simulink model "VB_RIFKF_GNSS_INS25"  (R2023a)
settings: Solver=FixedStepAuto  StartTime=0  StopTime=500  FixedStep=0.01  RelTol=1e-3
InitFcn:
  | resilient_initNavigation1216;
  | init_param;
undefined symbols (not defined in the file or in its folder): dt, g0, gam0_rad, ISUS_flag, magnitude, p, P0, P0_RIEKF, param, pd0, pe0, phi0_rad, pn0, psi, psi0_rad, state_dim, vd0, ve0, vn0
libraries: simulink_extras x68, dspstat3 x54, sharedtransform x47, simulink x43, matrix_library x9, sharedTrackingLibrary x5, dspfactors x4, aerolibconvert2 x3, aerolibtransform2 x3
(part 21 of 22)

== matlab function VB_RIFKF_GNSS_INS25/No.1_Sensor_Data_Process1/Magn_Data_Process/MATLAB Function1 ==
  data: u input; y output
function y = Normalization(u)
   dim = 3;
   y = zeros(dim,1);
y = double(u/sqrt(u(1)^2 + u(2)^2 + u(3)^2));

== matlab function VB_RIFKF_GNSS_INS25/No.1_Sensor_Data_Process1/Magn_Data_Process/Magn_preprocessing/MATLAB Function1 ==
  data: curr_input input single; curr_output output single; sample_freq input single; cutoff_freq input single
function curr_output = second_LPF_Butter_x(curr_input,sample_freq,cutoff_freq)
   persistent input_x;
   persistent output_x;

   if isempty(input_x)
       input_x = [0;0;0];
   end
   
   if isempty(output_x)
       output_x = [0;0;0];
   end
    B = [0,0,0];
    A = [0,0,0];
    M_PI_F = 3.1415926;
	fr = sample_freq / cutoff_freq;
	ohm = tan( M_PI_F / fr );
	c = 1.0 + 2.0 * cos( M_PI_F / 4.0 ) * ohm + ohm * ohm;
	B(1) = ohm * ohm / c;
	B(2) = 2.0 * B(1);
	B(3) = B(1);
	A(1) = 2.0 * ( ohm * ohm - 1.0) / c;
	A(2) = (1.0 - 2.0 * cos( M_PI_F / 4.0 ) * ohm + ohm * ohm) / c;
	%/*获取最新输入*/
	input_x(3) = curr_input;
	%/* Butterworth */
	output_x(3) =B(1) * input_x(3) + B(2) * input_x(2) +B(3) * input_x(1) - A(1) * output_x(2) - A(2) * output_x(1);
	curr_output = single(output_x(3));
   % /* 输入序列保存 */
	input_x(1) = input_x(2);
	input_x(2) = input_x(3);
	%/*输出序列保存 */
	output_x(1) = output_x(2);
	output_x(2) = output_x(3);

== matlab function VB_RIFKF_GNSS_INS25/No.1_Sensor_Data_Process1/Magn_Data_Process/Magn_preprocessing/MATLAB Function2 ==
  data: curr_input input single; curr_output output single; sample_freq input single; cutoff_freq input single
function curr_output = second_LPF_Butter_x(curr_input,sample_freq,cutoff_freq)
   persistent input_x;
   persistent output_x;

   if isempty(input_x)
       input_x = [0;0;0];
   end
   
   if isempty(output_x)
       output_x = [0;0;0];
   end
    B = [0,0,0];
    A = [0,0,0];
    M_PI_F = 3.1415926;
	fr = sample_freq / cutoff_freq;
	ohm = tan( M_PI_F / fr );
	c = 1.0 + 2.0 * cos( M_PI_F / 4.0 ) * ohm + ohm * ohm;
	B(1) = ohm * ohm / c;
	B(2) = 2.0 * B(1);
	B(3) = B(1);
	A(1) = 2.0 * ( ohm * ohm - 1.0) / c;
	A(2) = (1.0 - 2.0 * cos( M_PI_F / 4.0 ) * ohm + ohm * ohm) / c;
	%/*获取最新输入*/
	input_x(3) = curr_input;
	%/* Butterworth */
	output_x(3) =B(1) * input_x(3) + B(2) * input_x(2) +B(3) * input_x(1) - A(1) * output_x(2) - A(2) * output_x(1);
	curr_output = single(output_x(3));
   % /* 输入序列保存 */
	input_x(1) = input_x(2);
	input_x(2) = input_x(3);
	%/*输出序列保存 */
	output_x(1) = output_x(2);
	output_x(2) = output_x(3);

== matlab function VB_RIFKF_GNSS_INS25/No.1_Sensor_Data_Process1/Magn_Data_Process/Magn_preprocessing/MATLAB Function3 ==
  data: curr_input input single; curr_output output single; sample_freq input single; cutoff_freq input single
function curr_output = second_LPF_Butter_x(curr_input,sample_freq,cutoff_freq)
   persistent input_x;
   persistent output_x;

   if isempty(input_x)
       input_x = [0;0;0];
   end
   
   if isempty(output_x)
       output_x = [0;0;0];
   end
    B = [0,0,0];
    A = [0,0,0];
    M_PI_F = 3.1415926;
	fr = sample_freq / cutoff_freq;
	ohm = tan( M_PI_F / fr );
	c = 1.0 + 2.0 * cos( M_PI_F / 4.0 ) * ohm + ohm * ohm;
	B(1) = ohm * ohm / c;
	B(2) = 2.0 * B(1);
	B(3) = B(1);
	A(1) = 2.0 * ( ohm * ohm - 1.0) / c;
	A(2) = (1.0 - 2.0 * cos( M_PI_F / 4.0 ) * ohm + ohm * ohm) / c;
	%/*获取最新输入*/
	input_x(3) = curr_input;
	%/* Butterworth */
	output_x(3) =B(1) * input_x(3) + B(2) * input_x(2) +B(3) * input_x(1) - A(1) * output_x(2) - A(2) * output_x(1);
	curr_output =single(output_x(3));
   % /* 输入序列保存 */
	input_x(1) = input_x(2);
	input_x(2) = input_x(3);
	%/*输出序列保存 */
	output_x(1) = output_x(2);
	output_x(2) = output_x(3);

== matlab function VB_RIFKF_GNSS_INS25/No.1_Sensor_Data_Process1/Subsystem/TD_baro/MATLAB Function2 ==
  data: T input single; u1 output; u0 input; u1 input single; u2 input single; h input single; r input single; u2 output
function [u1,u2]=diff_TD_2(T,u0,u1,u2,h,r)
    %init
    %T是信号周期，u0原始信号输入，u1跟踪原始信号，u2原始信号差分值，
    %h滤波因子（h=T时接近一阶差分）越大滤波好延迟大；r速度因子，越大跟踪的越快但是噪声放大；

	x1=0; x2=0;
	delta=0;
	delta0=0;
	y=0;
	fabs_y=0;
	a0=0;
	a=0;
    fst=0;
    
	x1 = u1;
	x2 = u2;
	delta = r*h;
	delta0 = delta*h;
	y = x1 - u0 + h*x2;
	fabs_y = abs(y);   
	a0 = sqrt(delta*delta + 8 * r*fabs_y);
    
	if (fabs_y <= delta0)
		a = x2 + y / h;
    else
        a = x2 + 0.5*(a0 - delta)*sign(y);
    end
    
	if (abs(a) <= delta)
		fst = -r*a / delta;
    else
		fst = -r*sign(a);
    end
	u1 = single(x1 + T*x2); %计算跟踪信号
	u2 = single(x2 + T*fst); % 计算微分信号

== matlab function VB_RIFKF_GNSS_INS25/ISUS_RIEKF3/Error State Kalman Filter M3/MATLAB Function4 ==
  data: t input; u input; y output
function y = fcn(t,u)
if  t<300
    y = u;
elseif t<400 
    y = false;
else 
    y = u;
end

== matlab function VB_RIFKF_GNSS_INS25/No.1_Sensor_Data_Process1/TOF_Data_Process/TD_baro/MATLAB Function2 ==
  data: T input single; u1 output; u0 input; u1 input single; u2 input single; h input single; r input single; u2 output
function [u1,u2]=diff_TD_2(T,u0,u1,u2,h,r)
    %init
    %T是信号周期，u0原始信号输入，u1跟踪原始信号，u2原始信号差分值，
    %h滤波因子（h=T时接近一阶差分）越大滤波好延迟大；r速度因子，越大跟踪的越快但是噪声放大；

	x1=0; x2=0;
	delta=0;
	delta0=0;
	y=0;
	fabs_y=0;
	a0=0;
	a=0;
    fst=0;
    
	x1 = u1;
	x2 = u2;
	delta = r*h;
	delta0 = delta*h;
	y = x1 - u0 + h*x2;
	fabs_y = abs(y);   
	a0 = sqrt(delta*delta + 8 * r*fabs_y);
    
	if (fabs_y <= delta0)
		a = x2 + y / h;
    else
        a = x2 + 0.5*(a0 - delta)*sign(y);
    end
    
	if (abs(a) <= delta)
		fst = -r*a / delta;
    else
		fst = -r*sign(a);
    end
	u1 = single(x1 + T*x2); %计算跟踪信号
	u2 = single(x2 + T*fst); % 计算微分信号

== matlab function VB_RIFKF_GNSS_INS25/read FC1_/MATLAB Function ==
  data: dpsi input; y output
function y = wrap_dpsi(dpsi)
    if dpsi > 180
        dpsi = dpsi -360;
    elseif dpsi < -180
        dpsi = dpsi + 360;
    else 
        dpsi = dpsi;
    end
y = dpsi;

== matlab function VB_RIFKF_GNSS_INS25/No.1_Sensor_Data_Process1/baro_Data_Process/TD_baro/MATLAB Function2 ==
  data: T input single; u1 output; u0 input; u1 input single; u2 input single; h input single; r input single; u2 output
function [u1,u2]=diff_TD_2(T,u0,u1,u2,h,r)
    %init
    %T是信号周期，u0原始信号输入，u1跟踪原始信号，u2原始信号差分值，
    %h滤波因子（h=T时接近一阶差分）越大滤波好延迟大；r速度因子，越大跟踪的越快但是噪声放大；

	x1=0; x2=0;
	delta=0;
	delta0=0;
	y=0;
	fabs_y=0;
	a0=0;
	a=0;
    fst=0;
    
	x1 = u1;
	x2 = u2;
	delta = r*h;
	delta0 = delta*h;
	y = x1 - u0 + h*x2;
	fabs_y = abs(y);   
	a0 = sqrt(delta*delta + 8 * r*fabs_y);
    
	if (fabs_y <= delta0)
		a = x2 + y / h;
    else
        a = x2 + 0.5*(a0 - delta)*sign(y);
    end
    
	if (abs(a) <= delta)
		fst = -r*a / delta;
    else
		fst = -r*sign(a);
    end
	u1 = single(x1 + T*x2); %计算跟踪信号
	u2 = single(x2 + T*fst); % 计算微分信号

== matlab function VB_RIFKF_GNSS_INS25/ISUS_RIEKF3/Error State Kalman Filter M1/MATLAB Function4 ==
  data: t input; y output
function y = fcn(t)
if t<200 
    y = 0;
elseif t<300
    y=1;

elseif t<400
    y=0;
else 
    y=0;
end

end

== matlab function VB_RIFKF_GNSS_INS25/ISUS_RIEKF2/Error State Kalman Filter M1/Cal Q1/MATLAB Function1 ==
  data: Q output; dt input
function Q = fcn(dt)
    % G.block(0, 0, 3, 3) = -exp_so3(-w_hat * dt) * Jr_so3(-w_hat * dt) * dt;
    %    G.block(6, 3, 3, 3) = -R_Gtoi.transpose() * dt;
    %    G.block(3, 3, 3, 3) = -0.5 * R_Gtoi.transpose() * dt * dt;
    %    G.block(9, 6, 3, 3).setIdentity();
    %    G.block(12, 9, 3, 3).setIdentity();
    

    cov_dim = 12;
    Q = zeros(cov_dim,cov_dim);
%     noises_sigma_a_2 = 2.0000e-4^2;
%     noises_sigma_w_2 = 1.6968e-4^2;
%     noises_sigma_ab_2 = 3.0000e-4^2;
%     noises_sigma_wb_2 = 1.9393e-5^2;
    noises_sigma_a_2 = 0.001^2*1;
    %noises_sigma_w_2 = 0.0001^2;
    noises_sigma_w_2 = 0.00001^2;
    noises_sigma_ab_2 = 1.0000e-4^2*1;
    noises_sigma_wb_2 = 0.0002^2;
    % noises_sigma_mb_2 = 0.001^2;
    % noises_sigma_dtheta_2 = (1/57.3)^2;
    % noises_sigma_dwind_2 = 0.01^2;
    Q = diag([noises_sigma_w_2 / dt * ones(3,1); ...
                noises_sigma_a_2 / dt * ones(3,1); ...
                noises_sigma_wb_2 * dt * ones(3,1); ...
                noises_sigma_ab_2 * dt * ones(3,1); ...
                ]);
    

end

== matlab function VB_RIFKF_GNSS_INS25/read FC1_1/MATLAB Function ==
  data: dpsi input; y output
function y = wrap_dpsi(dpsi)
    if dpsi > 180
        dpsi = dpsi -360;
    elseif dpsi < -180
        dpsi = dpsi + 360;
    else 
        dpsi = dpsi;
    end
y = dpsi;

== matlab function VB_RIFKF_GNSS_INS25/No.1_Sensor_Data_Process2/GPS_Data_Process/LLA2NED/initGPSLLA ==
  data: QGCinitflag input; gpsLLA0_rad output; GPSfixtype input; gps_LLA_rad input; init_GPSLLAflag output
function [gpsLLA0_rad,init_GPSLLAflag] = initGPSLLA0(QGCinitflag,GPSfixtype,gps_LLA_rad)
    persistent initGPSLLAflag;
    persistent gpsLLA0;

    if isempty(initGPSLLAflag)
        initGPSLLAflag = 0;
    end
    if isempty(gpsLLA0)
        %初始GPS未进入定位状态，给定值
%          gpsLLA0 = [28.2/57.3;113/57.3;0];
        gpsLLA0 = zeros(3,1);
    end
    if (initGPSLLAflag == 0 && GPSfixtype >= 1) || (QGCinitflag == 1 && GPSfixtype >= 1)
        % 当GPS第一次初始化位置时，当GPSfixtype >=1 时，自动初始化一次位置，initGPSLLAflag置1
        % 或者是利用QGCinitflag地面站重新修正，不过需要满足GPSfixtype>=1的条件
        gpsLLA0 = gps_LLA_rad;
        initGPSLLAflag = 1;
    end
    gpsLLA0_rad = gpsLLA0;
    init_GPSLLAflag = initGPSLLAflag;
end

== matlab function VB_RIFKF_GNSS_INS25/No.1_Sensor_Data_Process2/IMU_Data_Process/accl_preprocessing2/MATLAB Function1 ==
  data: curr_input input; curr_output output single; sample_freq input; cutoff_freq input
function curr_output = second_LPF_Butter_x(curr_input,sample_freq,cutoff_freq)
   persistent input_x;
   persistent output_x;

   if isempty(input_x)
       input_x = [0;0;0];
   end
   
   if isempty(output_x)
       output_x = [0;0;0];
   end
    B = [0,0,0];
    A = [0,0,0];
    M_PI_F = 3.1415926;
	fr = sample_freq / cutoff_freq;
	ohm = tan( M_PI_F / fr );
	c = 1.0 + 2.0 * cos( M_PI_F / 4.0 ) * ohm + ohm * ohm;
	B(1) = ohm * ohm / c;
	B(2) = 2.0 * B(1);
	B(3) = B(1);
	A(1) = 2.0 * ( ohm * ohm - 1.0) / c;
	A(2) = (1.0 - 2.0 * cos( M_PI_F / 4.0 ) * ohm + ohm * ohm) / c;
	%/*获取最新输入*/
	input_x(3) = curr_input;
	%/* Butterworth */
	output_x(3) =B(1) * input_x(3) + B(2) * input_x(2) +B(3) * input_x(1) - A(1) * output_x(2) - A(2) * output_x(1);
	curr_output = single(output_x(3));
   % /* 输入序列保存 */
	input_x(1) = input_x(2);
	input_x(2) = input_x(3);
	%/*输出序列保存 */
	output_x(1) = output_x(2);
	output_x(2) = output_x(3);

== matlab function VB_RIFKF_GNSS_INS25/ISUS_RIEKF3/INS propogation1/att update/MATLAB Function ==
  data: Rbn_k_1 input; Rbn output; w input; dt input
function Rbn = fcn(Rbn_k_1, w, dt)
    Rbn =  Rbn_k_1 * exp_so3( w * dt);
end

== matlab function VB_RIFKF_GNSS_INS25/ISUS_RIEKF3/Error State Kalman Filter M1/VB-Extended Kalman Filter M2/Correct M1/MATLAB Function ==
  data: u input; y output
function y = fcn(u)

y = tril(u);

== matlab function VB_RIFKF_GNSS_INS25/No.1_Sensor_Data_Process2/IMU_Data_Process/accl_preprocessing2/MATLAB Function2 ==
  data: curr_input input; curr_output output single; sample_freq input; cutoff_freq input
function curr_output = second_LPF_Butter_x(curr_input,sample_freq,cutoff_freq)
   persistent input_x;
   persistent output_x;

   if isempty(input_x)
       input_x = [0;0;0];
   end
   
   if isempty(output_x)
       output_x = [0;0;0];
   end
    B = [0,0,0];
    A = [0,0,0];
    M_PI_F = 3.1415926;
	fr = sample_freq / cutoff_freq;
	ohm = tan( M_PI_F / fr );
	c = 1.0 + 2.0 * cos( M_PI_F / 4.0 ) * ohm + ohm * ohm;
	B(1) = ohm * ohm / c;
	B(2) = 2.0 * B(1);
	B(3) = B(1);
	A(1) = 2.0 * ( ohm * ohm - 1.0) / c;
	A(2) = (1.0 - 2.0 * cos( M_PI_F / 4.0 ) * ohm + ohm * ohm) / c;
	%/*获取最新输入*/
	input_x(3) = curr_input;
	%/* Butterworth */
	output_x(3) =B(1) * input_x(3) + B(2) * input_x(2) +B(3) * input_x(1) - A(1) * output_x(2) - A(2) * output_x(1);
	curr_output = single(output_x(3));
   % /* 输入序列保存 */
	input_x(1) = input_x(2);
	input_x(2) = input_x(3);
	%/*输出序列保存 */
	output_x(1) = output_x(2);
	output_x(2) = output_x(3);

== matlab function VB_RIFKF_GNSS_INS25/No.1_Sensor_Data_Process2/IMU_Data_Process/accl_preprocessing2/MATLAB Function3 ==
  data: curr_input input; curr_output output single; sample_freq input; cutoff_freq input
function curr_output = second_LPF_Butter_x(curr_input,sample_freq,cutoff_freq)
   persistent input_x;
   persistent output_x;

   if isempty(input_x)
       input_x = [0;0;0];
   end
   
   if isempty(output_x)
       output_x = [0;0;0];
   end
    B = [0,0,0];
    A = [0,0,0];
    M_PI_F = 3.1415926;
	fr = sample_freq / cutoff_freq;
	ohm = tan( M_PI_F / fr );
	c = 1.0 + 2.0 * cos( M_PI_F / 4.0 ) * ohm + ohm * ohm;
	B(1) = ohm * ohm / c;
	B(2) = 2.0 * B(1);
	B(3) = B(1);
	A(1) = 2.0 * ( ohm * ohm - 1.0) / c;
	A(2) = (1.0 - 2.0 * cos( M_PI_F / 4.0 ) * ohm + ohm * ohm) / c;
	%/*获取最新输入*/
	input_x(3) = curr_input;
	%/* Butterworth */
	output_x(3) =B(1) * input_x(3) + B(2) * input_x(2) +B(3) * input_x(1) - A(1) * output_x(2) - A(2) * output_x(1);
	curr_output = single(output_x(3));
   % /* 输入序列保存 */
	input_x(1) = input_x(2);
	input_x(2) = input_x(3);
	%/*输出序列保存 */
	output_x(1) = output_x(2);
	output_x(2) = output_x(3);

== matlab function VB_RIFKF_GNSS_INS25/No.1_Sensor_Data_Process2/IMU_Data_Process/gyro_preprocessing2/MATLAB Function1 ==
  data: curr_input input single; curr_output output single; sample_freq input single; cutoff_freq input single
function curr_output = second_LPF_Butter_x(curr_input,sample_freq,cutoff_freq)
   persistent input_x;
   persistent output_x;

   if isempty(input_x)
       input_x = [0;0;0];
   end
   
   if isempty(output_x)
       output_x = [0;0;0];
   end
    B = [0,0,0];
    A = [0,0,0];
    M_PI_F = 3.1415926;
	fr = sample_freq / cutoff_freq;
	ohm = tan( M_PI_F / fr );
	c = 1.0 + 2.0 * cos( M_PI_F / 4.0 ) * ohm + ohm * ohm;
	B(1) = ohm * ohm / c;
	B(2) = 2.0 * B(1);
	B(3) = B(1);
	A(1) = 2.0 * ( ohm * ohm - 1.0) / c;
	A(2) = (1.0 - 2.0 * cos( M_PI_F / 4.0 ) * ohm + ohm * ohm) / c;
	%/*获取最新输入*/
	input_x(3) = curr_input;
	%/* Butterworth */
	output_x(3) =B(1) * input_x(3) + B(2) * input_x(2) +B(3) * input_x(1) - A(1) * output_x(2) - A(2) * output_x(1);
	curr_output = single(output_x(3));
   % /* 输入序列保存 */
	input_x(1) = input_x(2);
	input_x(2) = input_x(3);
	%/*输出序列保存 */
	output_x(1) = output_x(2);
	output_x(2) = output_x(3);

== matlab function VB_RIFKF_GNSS_INS25/ISUS_RIEKF3/Error State Kalman Filter M1/VB-Extended Kalman Filter M2/Correct M1/Subsystem2/MATLAB Function1 ==
  data: u input; y output; X input; ISUS_flag input
function y = fcn(u, X, ISUS_flag)
if ISUS_flag == 0
    y = X;
else
     y = u;
    %y(1:9,1:9) = u;
end

== matlab function VB_RIFKF_GNSS_INS25/ISUS_RIEKF3/Error State Kalman Filter M1/VB-Extended Kalman Filter M2/Correct M1/innovation calculation/MATLAB Function ==
  data: u input; y output
function y = fcn(u)

y = u*u';

== matlab function VB_RIFKF_GNSS_INS25/ISUS_RIEKF3/Error State Kalman Filter M1/VB-Extended Kalman Filter M2/Output/MATLAB Function ==
  data: S input; P output
function P = fcn(S)
    
    % Get back Covariance from Square-root Covariance
    P = S*S';
    %P = 1/2*(S+S');
    
end

== matlab function VB_RIFKF_GNSS_INS25/No.1_Sensor_Data_Process2/IMU_Data_Process/gyro_preprocessing2/MATLAB Function2 ==
  data: curr_input input single; curr_output output single; sample_freq input single; cutoff_freq input single
function curr_output = second_LPF_Butter_x(curr_input,sample_freq,cutoff_freq)
   persistent input_x;
   persistent output_x;

   if isempty(input_x)
       input_x = [0;0;0];
   end
   
   if isempty(output_x)
       output_x = [0;0;0];
   end
    B = [0,0,0];
    A = [0,0,0];
    M_PI_F = 3.1415926;
	fr = sample_freq / cutoff_freq;
	ohm = tan( M_PI_F / fr );
	c = 1.0 + 2.0 * cos( M_PI_F / 4.0 ) * ohm + ohm * ohm;
	B(1) = ohm * ohm / c;
	B(2) = 2.0 * B(1);
	B(3) = B(1);
	A(1) = 2.0 * ( ohm * ohm - 1.0) / c;
	A(2) = (1.0 - 2.0 * cos( M_PI_F / 4.0 ) * ohm + ohm * ohm) / c;
	%/*获取最新输入*/
	input_x(3) = curr_input;
	%/* Butterworth */
	output_x(3) =B(1) * input_x(3) + B(2) * input_x(2) +B(3) * input_x(1) - A(1) * output_x(2) - A(2) * output_x(1);
	curr_output = single(output_x(3));
   % /* 输入序列保存 */
	input_x(1) = input_x(2);
	input_x(2) = input_x(3);
	%/*输出序列保存 */
	output_x(1) = output_x(2);
	output_x(2) = output_x(3);

== matlab function VB_RIFKF_GNSS_INS25/ISUS_RIEKF3/Error State Kalman Filter M1/VB-Extended Kalman Filter M2/Predict/Predict ==
  settings: updateMethod=DISCRETE  sampleTime=SampleTime
  data: x input; xNew output; P input; Q input; uState input; unused input; P output; pS parameter
function [xNew,P] = fcn(x,P,Q,uState,~,pS)
% ekfCorrect Prediction step for EKF
%
%   Copyright 2016-2021 The MathWorks, Inc.

%#codegen

% If process noise is time-varying then compute square-root
% factorization.
if pS.HasTimeVaryingQ
   Q = matlabshared.tracking.internal.svdPSD(Q);
end

% Construct fcn handles
if pS.IsSimulinkFcn
    StateTransitionJacobianFcnH_SL = str2func(pS.FcnName);
    if pS.HasAdditiveNoise
        StateTransitionFcnH = @(fState)StateTransitionJacobianFcnH_SL(fState);
    else
        StateTransitionFcnH = @(fState,fProcNoise)StateTransitionJacobianFcnH_SL(fState,fProcNoise);
    end
else
    StateTransitionFcnH = str2func(pS.FcnName);
end
if pS.HasJacobian
    if pS.IsSimulinkFcn
        StateTransitionJacobianFcnH_SL = str2func(pS.JacobianFcnName);
        if pS.HasAdditiveNoise
            StateTransitionJacobianFcnH = @(fState)StateTransitionJacobianFcnH_SL(fState);
        else
            StateTransitionJacobianFcnH = @(fState,fProcNoise)StateTransitionJacobianFcnH_SL(fState,fProcNoise);
        end
    else
        StateTransitionJacobianFcnH = str2func(pS.JacobianFcnName);
    end
else
    StateTransitionJacobianFcnH = [];
end

switch pS.NumberOfExtraArgumentInports
    case 0
        extraArgs = {};
    case 1
        extraArgs = {uState};
    otherwise
        assert(false);
end

% Check if dimensions and type of State and Jacobian are correct
if pS.HasAdditiveNoise
   % Additive noise
   
   % StateTransitionFcn
   xTry = StateTransitionFcnH(x, extraArgs{:});
   
   if pS.IsSimulinkFcn
      hasError = any(size(x) ~= size(xTry));
   else
      hasError = any(size(x) ~= size(xTry)) || ~isa(xTry, class(x));
   end
   
   coder.internal.errorIf(...
      hasError,...
      'shared_tracking:ExtendedKalmanFilter:StateNonMatchingSizeOrClass',...
      'StateTransitionFcn', 'State', numel(x));
   
   if pS.HasJacobian
      % Jacobian
      F = StateTransitionJacobianFcnH(x, extraArgs{:});
      % F needs to be square
      isSizeNotCorrect = ~all(size(F) == numel(x));
      
      if pS.IsSimulinkFcn
         hasError = isSizeNotCorrect;
      else
         hasError = isSizeNotCorrect || ~isa(F, class(x));
      end
      
      coder.internal.errorIf(...
         hasError,...
         'shared_tracking:ExtendedKalmanFilter:StateTransitionJacobianNonMatchingSizeOrClass',...
         'StateTransitionJacobianFcn', numel(x));
   end
else
   % Non-additive noise
   
   % StateTransitionFcn
   xTry = StateTransitionFcnH(x, zeros(size(Q,1),1,'like',x),extraArgs{:});
   
   if pS.IsSimulinkFcn
      hasError = any(size(x) ~= size(xTry));
   else
      hasError = any(size(x) ~= size(xTry)) || ~isa(xTry, class(x));
   end
   
   coder.internal.errorIf(...
      hasError,...
      'shared_tracking:ExtendedKalmanFilter:StateNonMatchingSizeOrClass',...
      'StateTransitionFcn', 'State', numel(x))
   
   if pS.HasJacobian
      % Jacobian
      F = StateTransitionJacobianFcnH(x, zeros(size(Q,1),1,'like',x),extraArgs{:});
      % F needs to be square
      isSizeNotCorrect = ~all(size(F) == numel(x));
      
      if pS.IsSimulinkFcn
         hasError = isSizeNotCorrect;
      else
         hasError = isSizeNotCorrect || ~isa(F, class(x));
      end
       
      coder.internal.errorIf(...
         hasError,...
         'shared_tracking:ExtendedKalmanFilter:StateTransitionJacobianNonMatchingSizeOrClass',...
         'StateTransitionJacobianFcn', numel(x));
   end
end

xNew = zeros(size(x),'like',x); %#ok<PREALL>

if pS.HasAdditiveNoise
    [xNew,P] = matlabshared.tracking.internal.EKFPredictorAdditive.predict(...
        Q,x,P,StateTransitionFcnH,StateTransitionJacobianFcnH,extraArgs{:});
else    
    [xNew,P] = matlabshared.tracking.internal.EKFPredictorNonAdditive.predict(...
        Q,x,P,StateTransitionFcnH,StateTransitionJacobianFcnH,extraArgs{:});
end
end

== matlab function VB_RIFKF_GNSS_INS25/read FC1_/Subsystem/MATLAB Function ==
  data: u input; y output; u_1 input
function y = fcn(u,u_1)
if abs(u) > 100
    y = u_1;
end
y = u;

== matlab function VB_RIFKF_GNSS_INS25/No.1_Sensor_Data_Process2/IMU_Data_Process/gyro_preprocessing2/MATLAB Function3 ==
  data: curr_input input single; curr_output output single; sample_freq input single; cutoff_freq input single
function curr_output = second_LPF_Butter_x(curr_input,sample_freq,cutoff_freq)
   persistent input_x;
   persistent output_x;

   if isempty(input_x)
       input_x = [0;0;0];
   end
   
   if isempty(output_x)
       output_x = [0;0;0];
   end
    B = [0,0,0];
    A = [0,0,0];
    M_PI_F = 3.1415926;
	fr = sample_freq / cutoff_freq;
	ohm = tan( M_PI_F / fr );
	c = 1.0 + 2.0 * cos( M_PI_F / 4.0 ) * ohm + ohm * ohm;
	B(1) = ohm * ohm / c;
	B(2) = 2.0 * B(1);
	B(3) = B(1);
	A(1) = 2.0 * ( ohm * ohm - 1.0) / c;
	A(2) = (1.0 - 2.0 * cos( M_PI_F / 4.0 ) * ohm + ohm * ohm) / c;
	%/*获取最新输入*/
	input_x(3) = curr_input;
	%/* Butterworth */
	output_x(3) =B(1) * input_x(3) + B(2) * input_x(2) +B(3) * input_x(1) - A(1) * output_x(2) - A(2) * output_x(1);
	curr_output = single(output_x(3));
   % /* 输入序列保存 */
	input_x(1) = input_x(2);
	input_x(2) = input_x(3);
	%/*输出序列保存 */
	output_x(1) = output_x(2);
	output_x(2) = output_x(3);

== matlab function VB_RIFKF_GNSS_INS25/ISUS_RIEKF3/INS propogation1/att update/MATLAB Function2 ==
  data: delta input; Rbn_correct output single size=[3,3]; Rbn input
function Rbn_correct = fcn(delta, Rbn)
    Rbn_correct = zeros(3,3);
     Rbn_correct = exp_so3(delta)* Rbn;
    %Rbn_correct =( eye(3) + skewMat(delta))* Rbn;
end

== matlab function VB_RIFKF_GNSS_INS25/No.1_Sensor_Data_Process2/Magn_Data_Process/MATLAB Function1 ==
  data: u input; y output
function y = Normalization(u)
   dim = 3;
   y = zeros(dim,1);
y = double(u/sqrt(u(1)^2 + u(2)^2 + u(3)^2));

== matlab function VB_RIFKF_GNSS_INS25/No.1_Sensor_Data_Process2/Magn_Data_Process/Magn_preprocessing/MATLAB Function1 ==
  data: curr_input input single; curr_output output single; sample_freq input single; cutoff_freq input single
function curr_output = second_LPF_Butter_x(curr_input,sample_freq,cutoff_freq)
   persistent input_x;
   persistent output_x;

   if isempty(input_x)
       input_x = [0;0;0];
   end
   
   if isempty(output_x)
       output_x = [0;0;0];
   end
    B = [0,0,0];
    A = [0,0,0];
    M_PI_F = 3.1415926;
	fr = sample_freq / cutoff_freq;
	ohm = tan( M_PI_F / fr );
	c = 1.0 + 2.0 * cos( M_PI_F / 4.0 ) * ohm + ohm * ohm;
	B(1) = ohm * ohm / c;
	B(2) = 2.0 * B(1);
	B(3) = B(1);
	A(1) = 2.0 * ( ohm * ohm - 1.0) / c;
	A(2) = (1.0 - 2.0 * cos( M_PI_F / 4.0 ) * ohm + ohm * ohm) / c;
	%/*获取最新输入*/
	input_x(3) = curr_input;
	%/* Butterworth */
	output_x(3) =B(1) * input_x(3) + B(2) * input_x(2) +B(3) * input_x(1) - A(1) * output_x(2) - A(2) * output_x(1);
	curr_output = single(output_x(3));
   % /* 输入序列保存 */
	input_x(1) = input_x(2);
	input_x(2) = input_x(3);
	%/*输出序列保存 */
	output_x(1) = output_x(2);
	output_x(2) = output_x(3);

== matlab function VB_RIFKF_GNSS_INS25/ISUS_RIEKF2/Error State Kalman Filter M1/Extended Kalman Filter M1/Correct M1/Correct ==
  settings: updateMethod=DISCRETE  sampleTime=SampleTime
  data: x input; xNew output; P input; P output; yMeas input; R input; uMeas input; blockOrdering input; pM parameter; blockOrdering output
function [xNew,P,blockOrdering] = fcn(x,P,yMeas,R,uMeas,blockOrdering,pM)
% ekfCorrect Correction step for EKF
%
%   Copyright 2016-2021 The MathWorks, Inc.

%#codegen

% If measurement noise is time-varying then compute square-root
% factorization.
if pM.HasTimeVaryingR
   R = matlabshared.tracking.internal.svdPSD(R);
end

% Construct the function handle for measurement fcn
if pM.IsSimulinkFcn
    MeasurementFcnH_SL = str2func(pM.FcnName);
    if pM.HasAdditiveNoise
        MeasurementFcnH = @(fState)MeasurementFcnH_SL(fState);
    else
        MeasurementFcnH = @(fState,fMeasNoise)MeasurementFcnH_SL(fState,fMeasNoise);
    end
else
    MeasurementFcnH = str2func(pM.FcnName);
end

% Construct the function handle for measurement Jacobian fcn
if pM.HasJacobian
    if pM.IsSimulinkFcn
        MeasurementJacobianFcnH_SL = str2func(pM.JacobianFcnName);
        if pM.HasAdditiveNoise
            MeasurementJacobianFcnH = @(fState)MeasurementJacobianFcnH_SL(fState);
        else
            MeasurementJacobianFcnH = @(fState,fMeasNoise)MeasurementJacobianFcnH_SL(fState,fMeasNoise);
        end
    else
        MeasurementJacobianFcnH = str2func(pM.JacobianFcnName);
    end
else
    MeasurementJacobianFcnH = [];
end

% Handle (optional) extra input arguments of the measurement & jacobian fcns
switch pM.NumberOfExtraArgumentInports
    case 0
        extraArgs = {};
    case 1
        extraArgs = {uMeas};
    otherwise
        assert(false);
end

% Construct the corrector, perform the update
if pM.HasAdditiveNoise
    ekfCorrector = matlabshared.tracking.internal.EKFCorrectorAdditive();
else
    ekfCorrector = matlabshared.tracking.internal.EKFCorrectorNonAdditive();
end

% Check if dimensions and type of Measurement and Jacobian are correct
if pM.HasAdditiveNoise
   % Additive noise
   
   % MeasurementFcn
   ztry = MeasurementFcnH(x, extraArgs{:});
   
   if pM.IsSimulinkFcn
      hasError = (numel(ztry) ~= numel(yMeas));
   else
      hasError = (numel(ztry) ~= numel(yMeas)) || ~isa(ztry, class(x));
   end
   
   coder.internal.errorIf(...
      hasError,...
      'shared_tracking:ExtendedKalmanFilter:MeasurementNonMatchingSizeOrClass',...
      'MeasurementFcn');
   
   if pM.HasJacobian
      % MeasurementJacobianFcn
      Htry = MeasurementJacobianFcnH(x, extraArgs{:});
      isSizeNotCorrect = numel(yMeas) ~= size(Htry,1) || numel(x) ~= size(Htry,2);
      
      if pM.IsSimulinkFcn
         hasError = isSizeNotCorrect;
      else
         hasError = isSizeNotCorrect || ~isa(Htry, class(x));
      end
      
      coder.internal.errorIf(...
         hasError,...
         'shared_tracking:ExtendedKalmanFilter:MeasurementJacobianNonMatchingSizeOrClass',...
         'MeasurementJacobianFcn',numel(yMeas),numel(x));
   end   
else
   % Non-additive noise
   
   % MeasurementFcn
   ztry = MeasurementFcnH(...
      x, zeros(size(R,1),1,'like',x), ...
      extraArgs{:});   

   if pM.IsSimulinkFcn
      hasError = (numel(ztry) ~= numel(yMeas));
   else
      hasError = (numel(ztry) ~= numel(yMeas)) || ~isa(ztry, class(x));
   end
   
   coder.internal.errorIf(...
      hasError,...
      'shared_tracking:ExtendedKalmanFilter:MeasurementNonMatchingSizeOrClass',...
      'MeasurementFcn');
   
   if pM.HasJacobian
      % MeasurementJacobianFcn
      Htry = MeasurementJacobianFcnH(...
         x, zeros(size(R,1),1,'like',x), ...
         extraArgs{:});
      
      isSizeNotCorrect = numel(yMeas) ~= size(Htry,1) || numel(x) ~= size(Htry,2);     
      
      if pM.IsSimulinkFcn
         hasError = isSizeNotCorrect;
      else
         hasError = isSizeNotCorrect || ~isa(Htry, class(x));
      end
      
      coder.internal.errorIf(...
         hasError,...
         'shared_tracking:ExtendedKalmanFilter:MeasurementJacobianNonMatchingSizeOrClass',...
         'MeasurementJacobianFcn',numel(yMeas),numel(x));
   end
end
% Measurement wrapping
ekfCorrector.HasMeasurementWrapping = pM.HasWrapping;

xNew = zeros(size(x),'like',x); %#ok<PREALL>
% wk = 0;
[xNew,P] = ekfCorrector.correct(...
        yMeas,R,x,P,MeasurementFcnH,MeasurementJacobianFcnH,extraArgs{:});
end

== matlab function VB_RIFKF_GNSS_INS25/No.1_Sensor_Data_Process2/Magn_Data_Process/Magn_preprocessing/MATLAB Function2 ==
  data: curr_input input single; curr_output output single; sample_freq input single; cutoff_freq input single
function curr_output = second_LPF_Butter_x(curr_input,sample_freq,cutoff_freq)
   persistent input_x;
   persistent output_x;

   if isempty(input_x)
       input_x = [0;0;0];
   end
   
   if isempty(output_x)
       output_x = [0;0;0];
   end
    B = [0,0,0];
    A = [0,0,0];
    M_PI_F = 3.1415926;
	fr = sample_freq / cutoff_freq;
	ohm = tan( M_PI_F / fr );
	c = 1.0 + 2.0 * cos( M_PI_F / 4.0 ) * ohm + ohm * ohm;
	B(1) = ohm * ohm / c;
	B(2) = 2.0 * B(1);
	B(3) = B(1);
	A(1) = 2.0 * ( ohm * ohm - 1.0) / c;
	A(2) = (1.0 - 2.0 * cos( M_PI_F / 4.0 ) * ohm + ohm * ohm) / c;
	%/*获取最新输入*/
	input_x(3) = curr_input;
	%/* Butterworth */
	output_x(3) =B(1) * input_x(3) + B(2) * input_x(2) +B(3) * input_x(1) - A(1) * output_x(2) - A(2) * output_x(1);
	curr_output = single(output_x(3));
   % /* 输入序列保存 */
	input_x(1) = input_x(2);
	input_x(2) = input_x(3);
	%/*输出序列保存 */
	output_x(1) = output_x(2);
	output_x(2) = output_x(3);

== matlab function VB_RIFKF_GNSS_INS25/No.1_Sensor_Data_Process2/Magn_Data_Process/Magn_preprocessing/MATLAB Function3 ==
  data: curr_input input single; curr_output output single; sample_freq input single; cutoff_freq input single
function curr_output = second_LPF_Butter_x(curr_input,sample_freq,cutoff_freq)
   persistent input_x;
   persistent output_x;

   if isempty(input_x)
       input_x = [0;0;0];
   end
   
   if isempty(output_x)
       output_x = [0;0;0];
   end
    B = [0,0,0];
    A = [0,0,0];
    M_PI_F = 3.1415926;
	fr = sample_freq / cutoff_freq;
	ohm = tan( M_PI_F / fr );
	c = 1.0 + 2.0 * cos( M_PI_F / 4.0 ) * ohm + ohm * ohm;
	B(1) = ohm * ohm / c;
	B(2) = 2.0 * B(1);
	B(3) = B(1);
	A(1) = 2.0 * ( ohm * ohm - 1.0) / c;
	A(2) = (1.0 - 2.0 * cos( M_PI_F / 4.0 ) * ohm + ohm * ohm) / c;
	%/*获取最新输入*/
	input_x(3) = curr_input;
	%/* Butterworth */
	output_x(3) =B(1) * input_x(3) + B(2) * input_x(2) +B(3) * input_x(1) - A(1) * output_x(2) - A(2) * output_x(1);
	curr_output =single(output_x(3));
   % /* 输入序列保存 */
	input_x(1) = input_x(2);
	input_x(2) = input_x(3);
	%/*输出序列保存 */
	output_x(1) = output_x(2);
	output_x(2) = output_x(3);

== matlab function VB_RIFKF_GNSS_INS25/ISUS_RIEKF3/Error State Kalman Filter M1/VB-Extended Kalman Filter M2/innovation calculation/MATLAB Function ==
  data: u input; y output
function y = fcn(u)

y = u*u';

== matlab function VB_RIFKF_GNSS_INS25/No.1_Sensor_Data_Process2/Subsystem/TD_baro/MATLAB Function2 ==
  data: T input single; u1 output; u0 input; u1 input single; u2 input single; h input single; r input single; u2 output
function [u1,u2]=diff_TD_2(T,u0,u1,u2,h,r)
    %init
    %T是信号周期，u0原始信号输入，u1跟踪原始信号，u2原始信号差分值，
    %h滤波因子（h=T时接近一阶差分）越大滤波好延迟大；r速度因子，越大跟踪的越快但是噪声放大；

	x1=0; x2=0;
	delta=0;
	delta0=0;
	y=0;
	fabs_y=0;
	a0=0;
	a=0;
    fst=0;
    
	x1 = u1;
	x2 = u2;
	delta = r*h;
	delta0 = delta*h;
	y = x1 - u0 + h*x2;
	fabs_y = abs(y);   
	a0 = sqrt(delta*delta + 8 * r*fabs_y);
    
	if (fabs_y <= delta0)
		a = x2 + y / h;
    else
        a = x2 + 0.5*(a0 - delta)*sign(y);
    end
    
	if (abs(a) <= delta)
		fst = -r*a / delta;
    else
		fst = -r*sign(a);
    end
	u1 = single(x1 + T*x2); %计算跟踪信号
	u2 = single(x2 + T*fst); % 计算微分信号

== matlab function VB_RIFKF_GNSS_INS25/No.1_Sensor_Data_Process2/TOF_Data_Process/TD_baro/MATLAB Function2 ==
  data: T input single; u1 output; u0 input; u1 input single; u2 input single; h input single; r input single; u2 output
function [u1,u2]=diff_TD_2(T,u0,u1,u2,h,r)
    %init
    %T是信号周期，u0原始信号输入，u1跟踪原始信号，u2原始信号差分值，
    %h滤波因子（h=T时接近一阶差分）越大滤波好延迟大；r速度因子，越大跟踪的越快但是噪声放大；

	x1=0; x2=0;
	delta=0;
	delta0=0;
	y=0;
	fabs_y=0;
	a0=0;
	a=0;
    fst=0;
    
	x1 = u1;
	x2 = u2;
	delta = r*h;
	delta0 = delta*h;
	y = x1 - u0 + h*x2;
	fabs_y = abs(y);   
	a0 = sqrt(delta*delta + 8 * r*fabs_y);
    
	if (fabs_y <= delta0)
		a = x2 + y / h;
    else
        a = x2 + 0.5*(a0 - delta)*sign(y);
    end
    
	if (abs(a) <= delta)
		fst = -r*a / delta;
    else
		fst = -r*sign(a);
    end
	u1 = single(x1 + T*x2); %计算跟踪信号
	u2 = single(x2 + T*fst); % 计算微分信号

== matlab function VB_RIFKF_GNSS_INS25/ISUS_RIEKF3/INS propogation1/vel//pos update/pos update/MATLAB Function ==
  data: dtheta input; pos_correct output single; KFState_dp input; pos input
function pos_correct = fcn(dtheta, KFState_dp, pos)
    
     pos_correct =  KFState_dp + exp_so3(dtheta)*pos;
    %pos_correct = pos + KFState_dp - skewMat(pos)*dtheta;
    
end

== matlab function VB_RIFKF_GNSS_INS25/No.1_Sensor_Data_Process2/baro_Data_Process/TD_baro/MATLAB Function2 ==
  data: T input single; u1 output; u0 input; u1 input single; u2 input single; h input single; r input single; u2 output
function [u1,u2]=diff_TD_2(T,u0,u1,u2,h,r)
    %init
    %T是信号周期，u0原始信号输入，u1跟踪原始信号，u2原始信号差分值，
    %h滤波因子（h=T时接近一阶差分）越大滤波好延迟大；r速度因子，越大跟踪的越快但是噪声放大；

	x1=0; x2=0;
	delta=0;
	delta0=0;
	y=0;
	fabs_y=0;
	a0=0;
	a=0;
    fst=0;
    
	x1 = u1;
	x2 = u2;
	delta = r*h;
	delta0 = delta*h;
	y = x1 - u0 + h*x2;
	fabs_y = abs(y);   
	a0 = sqrt(delta*delta + 8 * r*fabs_y);
    
	if (fabs_y <= delta0)
		a = x2 + y / h;
    else
        a = x2 + 0.5*(a0 - delta)*sign(y);
    end
    
	if (abs(a) <= delta)
		fst = -r*a / delta;
    else
		fst = -r*sign(a);
    end
	u1 = single(x1 + T*x2); %计算跟踪信号
	u2 = single(x2 + T*fst); % 计算微分信号

== matlab function VB_RIFKF_GNSS_INS25/ISUS_RIEKF3/Error State Kalman Filter M1/VB-Extended Kalman Filter M2/Correct M1/Correct1 ==
  settings: updateMethod=DISCRETE  sampleTime=SampleTime
  data: x input; xNew output; P input; P output; yMeas input; R input; uMeas input; blockOrdering input; pM parameter; blockOrdering output; alfa input; beta input; N input; alfa output; beta output; H input; R_VB output; R output
function [xNew,P,blockOrdering,alfa,beta,R_VB,R] = fcn(x,P,yMeas,R,uMeas,blockOrdering,pM,alfa,beta, N, H)
% ekfCorrect Correction step for EKF
%,alfa,beta,N
% xNew=x;
rou = 0.99;
alfa = alfa+0.5;
alfa = rou*alfa;
beta = rou*beta;
betaBak = beta;
P_pre=P;
mk_Pre=x;
x_Pre=x;
z=yMeas;
%%%%%Time update
 % for i = 1:N
   R_VB = diag(sqrt(abs(beta./alfa)));
    % mk = mk_Pre+P_pre*H'*pinv(H*P_pre*H'+R_VB)*(z-H*mk_Pre);
    % P1 = P_pre-P_pre*H'*pinv(H*P_pre*H'+R_VB)*H*P_pre;
    % beta = betaBak+1/2*(z-H*mk).^2+1/2*diag(H*P*H');
    % K = P_pre*H'*pinv(H*P_pre*H'+R_VB);
    % x_VB = x_Pre+K*(z-H*x_Pre);
%   Copyright 2016-2021 The MathWorks, Inc.

%#codegen

% If measurement noise is time-varying then compute square-root
% factorization.
if pM.HasTimeVaryingR
   R = matlabshared.tracking.internal.svdPSD(R);
end

% Construct the function handle for measurement fcn
if pM.IsSimulinkFcn
    MeasurementFcnH_SL = str2func(pM.FcnName);
    if pM.HasAdditiveNoise
        MeasurementFcnH = @(fState)MeasurementFcnH_SL(fState);
    else
        MeasurementFcnH = @(fState,fMeasNoise)MeasurementFcnH_SL(fState,fMeasNoise);
    end
else
    MeasurementFcnH = str2func(pM.FcnName);
end

% Construct the function handle for measurement Jacobian fcn
if pM.HasJacobian
    if pM.IsSimulinkFcn
        MeasurementJacobianFcnH_SL = str2func(pM.JacobianFcnName);
        if pM.HasAdditiveNoise
            MeasurementJacobianFcnH = @(fState)MeasurementJacobianFcnH_SL(fState);
        else
            MeasurementJacobianFcnH = @(fState,fMeasNoise)MeasurementJacobianFcnH_SL(fState,fMeasNoise);
        end
    else
        MeasurementJacobianFcnH = str2func(pM.JacobianFcnName);
    end
else
    MeasurementJacobianFcnH = [];
end

% Handle (optional) extra input arguments of the measurement & jacobian fcns
switch pM.NumberOfExtraArgumentInports
    case 0
        extraArgs = {};
    case 1
        extraArgs = {uMeas};
    otherwise
        assert(false);
end

% Construct the corrector, perform the update
if pM.HasAdditiveNoise
    ekfCorrector = matlabshared.tracking.internal.EKFCorrectorAdditive();
else
    ekfCorrector = matlabshared.tracking.internal.EKFCorrectorNonAdditive();
end

% Check if dimensions and type of Measurement and Jacobian are correct
if pM.HasAdditiveNoise
   % Additive noise
   
   % MeasurementFcn
   ztry = MeasurementFcnH(x, extraArgs{:});
   
   if pM.IsSimulinkFcn
      hasError = (numel(ztry) ~= numel(yMeas));
   else
      hasError = (numel(ztry) ~= numel(yMeas)) || ~isa(ztry, class(x));
   end
   
   coder.internal.errorIf(...
      hasError,...
      'shared_tracking:ExtendedKalmanFilter:MeasurementNonMatchingSizeOrClass',...
      'MeasurementFcn');
   
   if pM.HasJacobian
      % MeasurementJacobianFcn
      Htry = MeasurementJacobianFcnH(x, extraArgs{:});
      isSizeNotCorrect = numel(yMeas) ~= size(Htry,1) || numel(x) ~= size(Htry,2);
      
      if pM.IsSimulinkFcn
         hasError = isSizeNotCorrect;
      else
         hasError = isSizeNotCorrect || ~isa(Htry, class(x));
      end
      
      coder.internal.errorIf(...
         hasError,...
         'shared_tracking:ExtendedKalmanFilter:MeasurementJacobianNonMatchingSizeOrClass',...
         'MeasurementJacobianFcn',numel(yMeas),numel(x));
   end   
else
   % Non-additive noise
   
   % MeasurementFcn
   ztry = MeasurementFcnH(...
      x, zeros(size(R,1),1,'like',x), ...
      extraArgs{:});   

   if pM.IsSimulinkFcn
      hasError = (numel(ztry) ~= numel(yMeas));
   else
      hasError = (numel(ztry) ~= numel(yMeas)) || ~isa(ztry, class(x));
   end
   
   coder.internal.errorIf(...
      hasError,...
      'shared_tracking:ExtendedKalmanFilter:MeasurementNonMatchingSizeOrClass',...
      'MeasurementFcn');
   
   if pM.HasJacobian
      % MeasurementJacobianFcn
      Htry = MeasurementJacobianFcnH(...
         x, zeros(size(R,1),1,'like',x), ...
         extraArgs{:});
      
      isSizeNotCorrect = numel(yMeas) ~= size(Htry,1) || numel(x) ~= size(Htry,2);     
      
      if pM.IsSimulinkFcn
         hasError = isSizeNotCorrect;
      else
         hasError = isSizeNotCorrect || ~isa(Htry, class(x));
      end
      
      coder.internal.errorIf(...
         hasError,...
         'shared_tracking:ExtendedKalmanFilter:MeasurementJacobianNonMatchingSizeOrClass',...
         'MeasurementJacobianFcn',numel(yMeas),numel(x));
   end
end
% Measurement wrapping
ekfCorrector.HasMeasurementWrapping = pM.HasWrapping;

xNew = zeros(size(x),'like',x); %#ok<PREALL>
% wk = 0;
[xNew,P] = ekfCorrector.correct(...
        yMeas,R,x,P,MeasurementFcnH,MeasurementJacobianFcnH,extraArgs{:});
%%
mk=xNew;
z=yMeas;
beta = betaBak+1/2*(z-H*mk).^2+1/2*diag(H*P*H');

%%
 % end
  
end

== matlab function VB_RIFKF_GNSS_INS25/ISUS_RIEKF3/Error State Kalman Filter M1/MATLAB Function3 ==
  data: t input; pos input; y1 output; y2 output; vel input
function [y1,y2] = fcn(t, pos, vel)
if t<200 
R1 = [0 0 0;0 0 0;0 0 0];
R2 = [0 0 0;0 0 0;0 0 0];

elseif t<300
    R1 = [10 0 0;0 10 0;0 0 10];
    R2 = [1 0 0;0 1 0;0 0 1];

elseif t<400
R1 = [0 0 0;0 0 0;0 0 0];
R2 = [0 0 0;0 0 0;0 0 0];


% R = (1+cos(pi*t))*R0;
else 
 % R1 = [100 0 0;0 100 0;0 0 100];
 %    R2 = [1 0 0;0 1 0;0 0 1];
R1 = [0 0 0;0 0 0;0 0 0];
R2 = [0 0 0;0 0 0;0 0 0];
end
SR1 = utchol(R1);
SR2 = utchol(R2);

y1=pos+SR1*randn(3,1);
y2=vel+SR2*randn(3,1);

end

== matlab function VB_RIFKF_GNSS_INS25/ER EKF/Error State Kalman Filter/MATLAB Function3 ==
  data: t input; pos input; P output; V output; vel input
function [P,V] = fcn(t, pos, vel)
if t<100
    R1 = [0 0 0;0 0 0;0 0 0];
    R2 = [0 0 0;0 0 0;0 0 0];

elseif   t<200 
    
R1 = (1+0.6*cos(pi*t))*[1 0 0;0 1 0;0 0 1]*10;
R2 = (1+0.6*cos(pi*t))*[1 0 0;0 1 0;0 0 1]*10;

elseif   t<300 

 R1 = [0 0 0;0 0 0;0 0 0];
 R2 = [0 0 0;0 0 0;0 0 0];

elseif t<400
    R1 = [10 0 0;0 10 0;0 0 10];
    R2 = [10 0 0;0 10 0;0 0 10];

else
    R1 = [0 0 0;0 0 0;0 0 0];
    R2 = [0 0 0;0 0 0;0 0 0];
end
SR1 = utchol(R1);
SR2 = utchol(R2);

P=pos+SR1*randn(3,1);
V=vel+SR2*randn(3,1);

end

== matlab function VB_RIFKF_GNSS_INS25/ISUS_RIEKF1/Error State Kalman Filter M1/Extended Kalman Filter M1/Correct M1/MATLAB Function ==
  data: R input; diagonal_elements output
function diagonal_elements = fcn(R)
diagonal_elements = diag(R);

== matlab function VB_RIFKF_GNSS_INS25/read FC1_/Subsystem1/MATLAB Function ==
  data: u input; y output; u_1 input
function y = fcn(u,u_1)
y = u;
if abs(u) > 100
    y = u_1;
end

== matlab function VB_RIFKF_GNSS_INS25/ER EKF/Error State Kalman Filter/Extended Kalman Filter1/Correct1/MATLAB Function ==
  data: R input; diagonal_elements output
function diagonal_elements = fcn(R)
diagonal_elements = diag(R);

== matlab function VB_RIFKF_GNSS_INS25/ISUS_RIEKF3/Error State Kalman Filter M1/MATLAB Function1 ==
  data: t input; pos input; y1 output; y2 output; vel input
function [y1,y2] = fcn(t, pos, vel)
if t<200 
R1 = [0 0 0;0 0 0;0 0 0];
R2 = [0 0 0;0 0 0;0 0 0];

elseif t<300
    R1 = [100 0 0;0 100 0;0 0 100];
    R2 = [1 0 0;0 1 0;0 0 1];

% R = (1+cos(pi*t))*R0;
else
R1 = [0 0 0;0 0 0;0 0 0];
R2 = [0 0 0;0 0 0;0 0 0];

end
SR1 = utchol(R1);
SR2 = utchol(R2);

y1=pos+SR1*randn(3,1);
y2=vel+SR2*randn(3,1);

end

== matlab function VB_RIFKF_GNSS_INS25/ISUS_RIEKF3/INS propogation1/vel//pos update/vel update/MATLAB Function ==
  data: dtheta input; vel_correct output single; KFState_dv input; vel input
function vel_correct = fcn(dtheta, KFState_dv, vel)
    
     vel_correct =  KFState_dv + exp_so3( dtheta)*vel;
    %vel_correct =  vel + KFState_dv - skewMat(vel)*dtheta;
end

== matlab function VB_RIFKF_GNSS_INS25/read FC1_/Subsystem2/MATLAB Function ==
  data: u input; y output; u_1 input
function y = fcn(u,u_1)
if abs(u) > 100
    y = u_1;
end
y = u;

== matlab function VB_RIFKF_GNSS_INS25/read FC1_y/MATLAB Function ==
  data: dpsi input; y output
function y = wrap_dpsi(dpsi)
    if dpsi > 180
        dpsi = dpsi -360;
    elseif dpsi < -180
        dpsi = dpsi + 360;
    else 
        dpsi = dpsi;
    end
y = dpsi;

== matlab function VB_RIFKF_GNSS_INS25/read FC1_y/Subsystem/MATLAB Function ==
  data: u input; y output; u_1 input
function y = fcn(u,u_1)
if abs(u) > 100
    y = u_1;
end
y = u;

== matlab function VB_RIFKF_GNSS_INS25/ISUS_RIEKF3/Error State Kalman Filter M1/Extended Kalman Filter M1/Correct M1/innovation calculation1/MATLAB Function ==
  data: u input; y output
function y = fcn(u)

y = u*u';

== matlab function VB_RIFKF_GNSS_INS25/ISUS_RIEKF3/Error State Kalman Filter M1/Extended Kalman Filter M1/Correct M1/innovation calculation1/MATLAB Function1 ==
  data: r input; beta output; S input; deltaV output
function [beta,deltaV] = fcn(r, S)
d=0.85;

k=trace(S);
deltaV = r/trace(S);

if deltaV <=d
    beta = d/abs(deltaV);
else
    beta=single(1);
end

== matlab function VB_RIFKF_GNSS_INS25/ISUS_RIEKF3/Error State Kalman Filter M1/Extended Kalman Filter M1/Correct M1/innovation calculation1/MATLAB Function3 ==
  data: r input; S input; Gamma output
function Gamma   = fcn(r, S)


Gamma = transpose(r)*inv(S)*r;

end

== matlab function VB_RIFKF_GNSS_INS25/read FC1_y/Subsystem1/MATLAB Function ==
  data: u input; y output; u_1 input
function y = fcn(u,u_1)
y = u;
if abs(u) > 100
    y = u_1;
end

== matlab function VB_RIFKF_GNSS_INS25/No.1_Sensor_Data_Process1/GPS_Data_Process/LLA2NED/MATLAB Function2 ==
  data: t input; u input; y output
function y = fcn(t,u)
if t<40
    s=1; 
    y = u;
elseif t<120 
    s=5; 
    y = u + (10*[0.05;0.05;0.01].*htwn(0.1,s,3));
elseif t<160 
    s=10; 
    y = u + (10*[0.05;0.05;0.01].*htwn(0.05,s,3));
else 
    s=20; 
    %y = u + ([0.05;0.05;0.01].*htwn(0.05,s,3));
    y = u
end

== matlab function VB_RIFKF_GNSS_INS25/ISUS_RIEKF1/Error State Kalman Filter M1/Cal Q1/MATLAB Function1 ==
  data: Q output; dt input
function Q = fcn(dt)
    % G.block(0, 0, 3, 3) = -exp_so3(-w_hat * dt) * Jr_so3(-w_hat * dt) * dt;
    %    G.block(6, 3, 3, 3) = -R_Gtoi.transpose() * dt;
    %    G.block(3, 3, 3, 3) = -0.5 * R_Gtoi.transpose() * dt * dt;
    %    G.block(9, 6, 3, 3).setIdentity();
    %    G.block(12, 9, 3, 3).setIdentity();
    

    cov_dim = 12;
    Q = zeros(cov_dim,cov_dim);
%     noises_sigma_a_2 = 2.0000e-4^2;
%     noises_sigma_w_2 = 1.6968e-4^2;
%     noises_sigma_ab_2 = 3.0000e-4^2;
%     noises_sigma_wb_2 = 1.9393e-5^2;
    noises_sigma_a_2 = 0.001^2*1;
    %noises_sigma_w_2 = 0.0001^2;
    noises_sigma_w_2 = 0.0001^2;
    noises_sigma_ab_2 = 1.0000e-4^2*1;
    noises_sigma_wb_2 = 0.0002^2;
    % noises_sigma_mb_2 = 0.001^2;
    % noises_sigma_dtheta_2 = (1/57.3)^2;
    % noises_sigma_dwind_2 = 0.01^2;
    Q = diag([noises_sigma_w_2 / dt * ones(3,1); ...
                noises_sigma_a_2 / dt * ones(3,1); ...
                noises_sigma_wb_2 * dt * ones(3,1); ...
                noises_sigma_ab_2 * dt * ones(3,1); ...
                ]);
    

end

== matlab function VB_RIFKF_GNSS_INS25/No.1_Sensor_Data_Process/GPS_Data_Process/LLA2NED/MATLAB Function2 ==
  data: t input; u input; y output
function y = fcn(t,u)
if t<100
    s=1; 
    y = u;
elseif t<160 
    s=5; 
    y = u + (10*[0.05;0.05;0.01].*htwn(0.1,s,3));
elseif t<260 
    s=10; 
    y = u + (10*[0.05;0.05;0.01].*htwn(0.05,s,3));
else 
    s=20; 
    %y = u + ([0.05;0.05;0.01].*htwn(0.05,s,3));
    y = u
end

== matlab function VB_RIFKF_GNSS_INS25/ISUS_RIEKF2/Error State Kalman Filter M1/Extended Kalman Filter M1/Output/MATLAB Function ==
  data: S input; P output
function P = fcn(S)
    
    % Get back Covariance from Square-root Covariance
    P = S*S';
    %P = 1/2*(S+S');
    
end

== matlab function VB_RIFKF_GNSS_INS25/ISUS_RIEKF3/INS propogation2/att update/MATLAB Function ==
  data: Rbn_k_1 input; Rbn output; w input; dt input
function Rbn = fcn(Rbn_k_1, w, dt)
    Rbn =  Rbn_k_1 * exp_so3( w * dt);
end
